simulink model "SemiOffline_DataImport_AND_Preprocessing_ECGandSCG3D"  (R2019a)
settings: Solver=FixedStepDiscrete  StartTime=0.0  StopTime=sim_time + param_frame_size_sec  FixedStep=1/fs  MaxStep=1/fs  RelTol=1e-3
undefined symbols (not defined in the file): fdesignblkfcn, fs, gcbh, param_frame_size_sec, tot_samples
(part 1 of 3)
settings Model: PacingRate=100  Creator=rcord  LastModifiedBy=rcord
settings SolverCC: ZeroCrossControl=DisableAll
settings DataIOCC: ExternalInput=[t, ecg, x, y, z]  LoadExternalInput=on  LoggingIntervals=[-inf,inf]

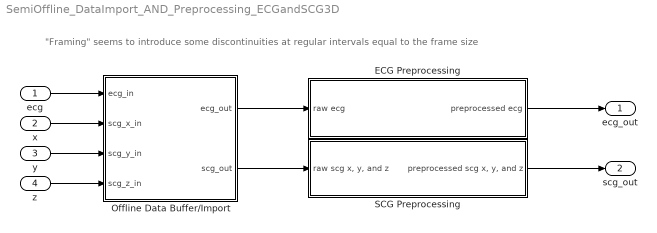
== system SemiOffline_DataImport_AND_Preprocessing_ECGandSCG3D ==
  note: "Framing" seems to introduce some discontinuities at regular intervals equal to the frame size
  ecg : Inport  SampleTime=1/fs
  x : Inport  Port=2  SampleTime=1/fs
  y : Inport  Port=3  SampleTime=1/fs
  z : Inport  Port=4  SampleTime=1/fs
  ECG Preprocessing : Subsystem  mask{param_ecg_gain_mv=1000, param_ecg_fc_lo=2.25, param_ecg_fc_hi=25, param_ecg_trans_bw=2}
      mask prompts: param_ecg_gain_mv "mV Conversion Gain"; param_ecg_fc_lo "Low Passband Frequency Corner (Hz)"; param_ecg_fc_hi "High Passband Frequency Corner (Hz)"; param_ecg_trans_bw "Transition bandwidth"
      mask init:
      | assignin('base','param_ecg_gain_mv',param_ecg_gain_mv)
      | assignin('base','param_ecg_fc_lo',param_ecg_fc_lo)
      | assignin('base','param_ecg_fc_hi',param_ecg_fc_hi)
      | assignin('base','param_ecg_trans_bw',param_ecg_trans_bw)
      mask DialogControl DescGroupVar Prompt: ECG Preprocessing
      mask DialogControl DescTextVar Prompt: Preprocessing of the ECG. This involves an amplificaiton stage followed by a filtfiltering operation (i.e. a front-back zero-phase FIR bandpass filter).
  Offline Data Buffer/Import : Subsystem  mask{param_frame_size_sec=15}
      mask prompts: param_frame_size_sec "Frame Size (in seconds)"
      mask init:
      | assignin('base','param_frame_size_sec',param_frame_size_sec)
      mask DialogControl DescGroupVar Prompt: Data Import Buffer
      mask DialogControl DescTextVar Prompt: The buffer size will specify the length of the jumping "frame" or "window". Subsequent analysis will be performed on each of these windows in succession.
  SCG Preprocessing : Subsystem  mask{param_scg_gain_mg=3333, param_scg_fc_lo=6, param_scg_fc_hi=37.5, param_scg_trans_bw=2.5}
      mask prompts: param_scg_gain_mg "V to mg Conversion Gain"; param_scg_fc_lo "Low Passband Frequency Corner (Hz)"; param_scg_fc_hi "High Passband Frequency Corner (Hz)"; param_scg_trans_bw "Transition bandwidth"
      mask init:
      | assignin('base','param_scg_gain_mg',param_scg_gain_mg)
      | assignin('base','param_scg_fc_lo',param_scg_fc_lo)
      | assignin('base','param_scg_fc_hi',param_scg_fc_hi)
      | assignin('base','param_scg_trans_bw',param_scg_trans_bw)
      mask DialogControl DescGroupVar Prompt: SCG Preprocessing
      mask DialogControl DescTextVar Prompt: Preprocessing of the SCG x, y, and z. The input is a single three-column vector containing the x, y, and z SCG components in its columns. The preprocessing involves an amplificaiton stage followed by a filtfiltering operation (i.e. a front-back zero-phase FIR bandpass filter). The filtering is identical for each of the three components.
  ecg_out : Outport
  scg_out : Outport  Port=2
  wires:
  ecg/1 -> Offline Data Buffer/Import/1(ecg_in)
  x/1 -> Offline Data Buffer/Import/2(scg_x_in)
  y/1 -> Offline Data Buffer/Import/3(scg_y_in)
  z/1 -> Offline Data Buffer/Import/4(scg_z_in)
  ECG Preprocessing/1(preprocessed ecg) -> ecg_out/1
  Offline Data Buffer/Import/1(ecg_out) -> ECG Preprocessing/1(raw ecg)
  Offline Data Buffer/Import/2(scg_out) -> SCG Preprocessing/1("raw scg x, y, and z")
  SCG Preprocessing/1("preprocessed scg x, y, and z") -> scg_out/1

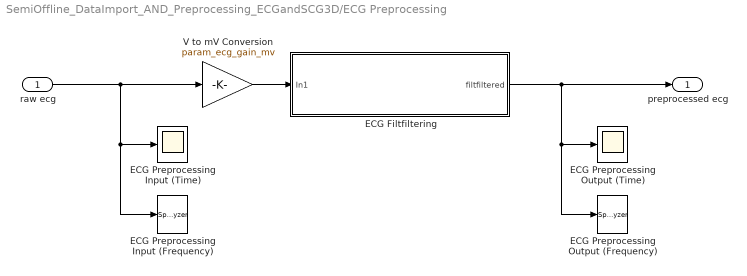
== system SemiOffline_DataImport_AND_Preprocessing_ECGandSCG3D/ECG Preprocessing ==
  raw ecg : Inport
  ECG Filtfiltering : Subsystem
  ECG Preprocessing Input (Frequency) : SpectrumAnalyzer
  ECG Preprocessing Input (Time) : Scope
  ECG Preprocessing Output (Frequency) : SpectrumAnalyzer
  ECG Preprocessing Output (Time) : Scope
  V to mV Conversion : Gain  Gain=param_ecg_gain_mv
  preprocessed ecg : Outport
  wires:
  ECG Filtfiltering/1(filtfiltered) -> preprocessed ecg/1, ECG Preprocessing Output (Time)/1, ECG Preprocessing Output (Frequency)/1
  raw ecg/1 -> ECG Preprocessing Input (Frequency)/1, ECG Preprocessing Input (Time)/1, V to mV Conversion/1
  V to mV Conversion/1 -> ECG Filtfiltering/1(In1)

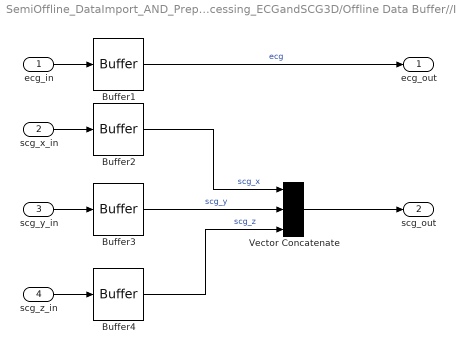
== system SemiOffline_DataImport_AND_Preprocessing_ECGandSCG3D/Offline Data Buffer//Import ==
  ecg_in : Inport
  scg_x_in : Inport  Port=2
  scg_y_in : Inport  Port=3
  scg_z_in : Inport  Port=4
  Buffer{1..4} (4 alike) : Buffer  N=param_frame_size_sec*fs  OutputFrames=off
  Vector Concatenate : Concatenate  NumInputs=3  Mode=Multidimensional array  ConcatenateDimension=2
  ecg_out : Outport
  scg_out : Outport  Port=2
  wires:
  ecg_in/1 -> Buffer1/1
  Buffer4/1 -> Vector Concatenate/3  "scg_z"
  Buffer2/1 -> Vector Concatenate/1  "scg_x"
  scg_x_in/1 -> Buffer2/1
  Vector Concatenate/1 -> scg_out/1
  Buffer1/1 -> ecg_out/1  "ecg"
  Buffer3/1 -> Vector Concatenate/2  "scg_y"
  scg_z_in/1 -> Buffer4/1
  scg_y_in/1 -> Buffer3/1

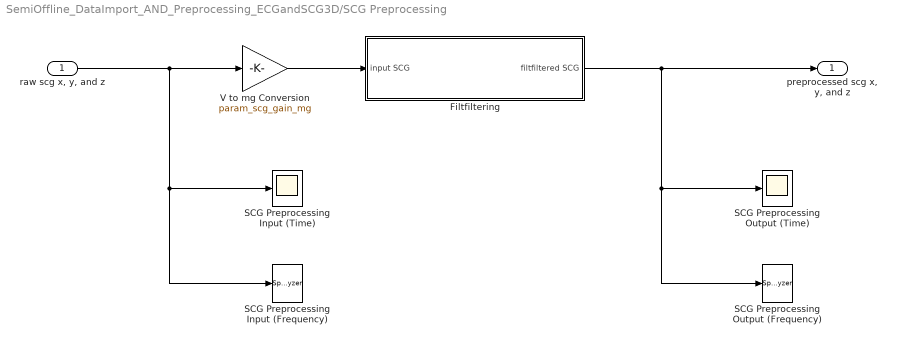
== system SemiOffline_DataImport_AND_Preprocessing_ECGandSCG3D/SCG Preprocessing ==
  "raw scg x, y, and z" : Inport
  Filtfiltering : Subsystem
  SCG Preprocessing Input (Frequency) : SpectrumAnalyzer
  SCG Preprocessing Input (Time) : Scope
  SCG Preprocessing Output (Frequency) : SpectrumAnalyzer
  SCG Preprocessing Output (Time) : Scope
  V to mg Conversion : Gain  Gain=param_scg_gain_mg
  "preprocessed scg x, y, and z" : Outport
  wires:
  V to mg Conversion/1 -> Filtfiltering/1(" input SCG")
  Filtfiltering/1(filtfiltered SCG) -> "preprocessed scg x, y, and z"/1, SCG Preprocessing Output (Frequency)/1, SCG Preprocessing Output (Time)/1
  "raw scg x, y, and z"/1 -> V to mg Conversion/1, SCG Preprocessing Input (Frequency)/1, SCG Preprocessing Input (Time)/1

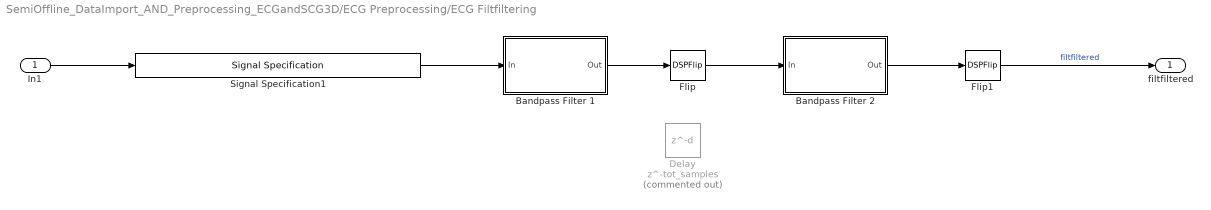
== system SemiOffline_DataImport_AND_Preprocessing_ECGandSCG3D/ECG Preprocessing/ECG Filtfiltering ==
  In1 : Inport
  Bandpass Filter 1 : Subsystem  DialogController=fdesignblkfcn  InitFcn=fdesignblkfcn(gcbh, {'InitFcn'});  mask(Bandpass Filter){}
      mask help: Design a bandpass filter
      settings: CopyFcn=fdesignblkfcn(gcbh, {'CopyFcn'});
      mask Help: helpview(mapfilelocation('dsp'), 'dspbandpassfilter');
      mask Display: disp('Bandpass');
  Bandpass Filter 2 : Subsystem  DialogController=fdesignblkfcn  InitFcn=fdesignblkfcn(gcbh, {'InitFcn'});  mask(Bandpass Filter){}
      mask help: Design a bandpass filter
      settings: CopyFcn=fdesignblkfcn(gcbh, {'CopyFcn'});
      mask Help: helpview(mapfilelocation('dsp'), 'dspbandpassfilter');
      mask Display: disp('Bandpass');
  Delay : Delay  Commented=on  DelayLength=tot_samples
  Flip : DSPFlip
  Flip1 : DSPFlip
  Signal Specification1 : SignalSpecification  Dimensions=[param_frame_size_sec*fs 1]  SampleTime=param_frame_size_sec
  filtfiltered : Outport
  wires:
  Flip/1 -> Bandpass Filter 2/1(In)
  Signal Specification1/1 -> Bandpass Filter 1/1(In)
  Flip1/1 -> filtfiltered/1  "filtfiltered"
  Bandpass Filter 1/1(Out) -> Flip/1
  In1/1 -> Signal Specification1/1
  Bandpass Filter 2/1(Out) -> Flip1/1

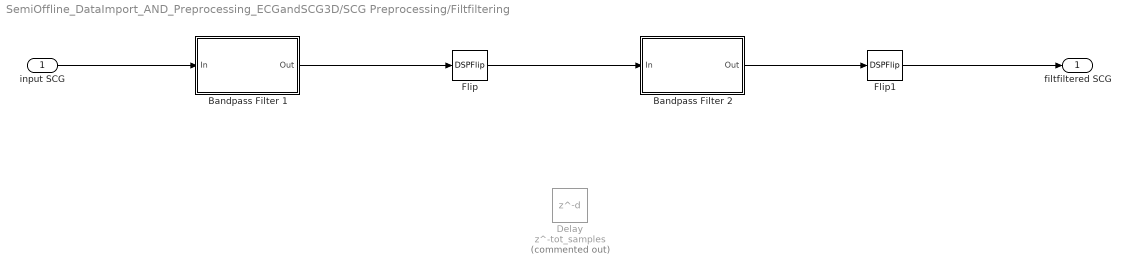
== system SemiOffline_DataImport_AND_Preprocessing_ECGandSCG3D/SCG Preprocessing/Filtfiltering ==
  " input SCG" : Inport
  Bandpass Filter 1 : Subsystem  DialogController=fdesignblkfcn  InitFcn=fdesignblkfcn(gcbh, {'InitFcn'});  mask(Bandpass Filter){}
      mask help: Design a bandpass filter
      settings: CopyFcn=fdesignblkfcn(gcbh, {'CopyFcn'});
      mask Help: helpview(mapfilelocation('dsp'), 'dspbandpassfilter');
      mask Display: disp('Bandpass');
  Bandpass Filter 2 : Subsystem  DialogController=fdesignblkfcn  InitFcn=fdesignblkfcn(gcbh, {'InitFcn'});  mask(Bandpass Filter){}
      mask help: Design a bandpass filter
      settings: CopyFcn=fdesignblkfcn(gcbh, {'CopyFcn'});
      mask Help: helpview(mapfilelocation('dsp'), 'dspbandpassfilter');
      mask Display: disp('Bandpass');
  Delay : Delay  Commented=on  DelayLength=tot_samples
  Flip : DSPFlip
  Flip1 : DSPFlip
  filtfiltered SCG : Outport
  wires:
  Bandpass Filter 2/1(Out) -> Flip1/1
  Bandpass Filter 1/1(Out) -> Flip/1
  Flip1/1 -> filtfiltered SCG/1
  " input SCG"/1 -> Bandpass Filter 1/1(In)
  Flip/1 -> Bandpass Filter 2/1(In)

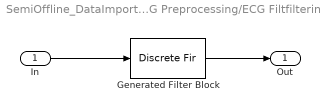
== system SemiOffline_DataImport_AND_Preprocessing_ECGandSCG3D/ECG Preprocessing/ECG Filtfiltering/Bandpass Filter 1 ==
  In : Inport
  Generated Filter Block : DiscreteFir  Tag=BlockMethodSubSystem  Coefficients=[0.000599681428480406667 0.00022427881711320835 0.000262189229493461906 0.000301151231840785058 0.000340510589773355293 0.000379471739139127223 0.000417264520068358531 0.000453028670626539611 0.000485966954942475358 0.00051520760979863558 0.000539947448272285867 0.000559296976009684673 0.000572459856652281327 0.000578602477107202379 0.000577082054079471073 0.000567310721348460796 0.000548962217988804477 0.000521740662199047796 0.000485547849092085506 0.000440237445712871403 0.000385936203776109077 0.0003229072755123711 0.000251933844194426903 0.000173864022162185553 8.96622951676985882e-05 -1.57244866912700784e-07 -9.44856236782579242e-05 -0.000191498736668446122 -0.000288821218832035532 -0.000387533990135975289 -0.000483387582565404498 -0.0005761939607201366 -0.000663970783304963915 -0.000744998643679979622 -0.000817872499416035523 -0.000880964362066854394 -0.000933038029693197195 -0.000972819175774386783 -0.000999391982786898819 -0.00101188643953785775 -0.00100975562147095736 -0.0009925777872959497 -0.000960301557973968888 -0.000913095371979611662 -0.000851475875971816542 -0.000776120817800070653 -0.000687956792167104684 -0.000588107835108653276 -0.000478027414632521848 -0.000359399960207810011 -0.000234020645553201104 -0.000103693767713263781 2.96347327928040449e-05 0.000163739535853423413 0.000296477349825991486 0.000425963905314958593 0.000550271710824708736 0.000666957213482007386 0.000774942628045007312 0.000872177327279355982 0.000957465516398583625 0.00102970621888984269 0.00108791155925947033 0.00113161169633735001 0.00116043044083965412 0.0011744928939702423 0.00117405121060814872 0.00115977134711482406 0.00113246741259064921 0.00109334691797877397 0.00104377213487224217 0.000985398948140998616 0.000919928026674857939 0.000849253670460306097 0.000775309012431770091 0.000700173020871669742 0.000625831434083841767 0.000554224460255208049 0.000487166253492989055 0.000426450533091061459 0.000373619349808891274 0.000329927391772101672 0.000296427775797514052 0.000274047129555466101 0.000263269264543539259 0.000264157227992290519 0.000276874450267364388 0.000300788149948878205 0.000335318317219354277 0.000379524997454130854 0.000432116465419417437 0.000491744413303003814 0.000556678027257966729 0.000625231365131872401 0.000695472120517187306 0.000765547328755601729 0.000833457105991844546 0.000897350978582148358 0.000955377677051596087 0.00100593089701688995 0.00104747392905528316 0.00107875626706505925 0.00109870509459187833 0.00110663185599915856 0.00110205240167736483 0.00108482227065854683 0.00105506279689406663 0.00101332829262456995 0.000960389758015832038 0.000897294817939977879 0.0008253500824062772 0.000746184239515585096 0.000661481098250255592 0.000573117805415166684 0.000483198626351262744 0.000393641448412858244 0.000306548825905859836 0.000223915957856876999 0.000147575494923837179 7.93483670767496796e-05 2.0679134117342313e-05 -2.70568547297773252e-05 -6.2900947686025382e-05 -8.60547436648419054e-05 -9.6171340327614761e-05 -9.31315796396773476e-05 -7.72460981475539256e-05 -4.90464702055338356e-05 -9.48878629550117885e-06 4.02424070543771421e-05 9.86143682268325855e-05 0.000163975772433438543 0.000234396831494164046 0.000307849569477817292 0.000382148726522325442 0.000455178453888958954 0.000524750281940376253 0.000588791425088850046 0.000645337762489050257 0.000692671840552972233 0.000729179983312047068 0.000753614641450886871 0.000765041942292764266 0.000762766365786752784 0.000746540173588745664 0.000716442000586304303 0.000672869753273410646 0.000616693112415834534 0.000548961839282761715 0.000471193538365353938 0.000385043306713752601 0.000292542948292242168 0.000195781895046972886 9.70798634232155033e-05 -1.26466659842236589e-06 -9.68248365214415734e-05 -0.000187315516146842245 -0.000270487917175212054 -0.000344346840215538515 -0.000407012200967724123 -0.000456962738277819839 -0.000492929167971300737 -0.000514057150433395722 -0.000519773775474877196 -0.000509999280888828277 -0.000484990084874355025 ...(+20204 chars)]  InputProcessing=Columns as channels (frame based)
  Out : Outport
  wires:
  In/1 -> Generated Filter Block/1
  Generated Filter Block/1 -> Out/1
